simulink model "offline_fuzzypid"  (R2015a)
settings: Solver=ode45  SolverMode=SingleTasking  StartTime=0.0  StopTime=10.0  RelTol=1e-3
libraries: fuzblock x1, simulink x1
settings Model: CovMetricSettings=dwe  CovHtmlReporting=off  covSaveCumulativeToWorkspaceVar=off  CovSaveSingleToWorkspaceVar=off  CovExternalEMLEnable=on  Creator=DwigHT  LastModifiedBy=DwigHT
settings DataIOCC: LimitDataPoints=off  SaveFormat=Dataset  ReturnWorkspaceOutputs=on
settings DebuggingCC: UnconnectedInputMsg=none  UnconnectedOutputMsg=none  UnconnectedLineMsg=none  SFUnexpectedBacktrackingDiag=error  SFNoUnconditionalDefaultTransitionDiag=error
settings HardwareCC: ProdBitPerPointer=64  ProdLargestAtomicFloat=Float  ProdIntDivRoundTo=Zero  ProdEndianess=LittleEndian  ProdHWDeviceType=Specified
settings ModelReferenceCC: PropagateSignalLabelsOutOfModel=on
settings SFSimCC: SimUseLocalCustomCode=on
settings RTWCC: RTWUseLocalCustomCode=on
settings GRTTargetCC: TargetLangStandard=C99 (ISO)

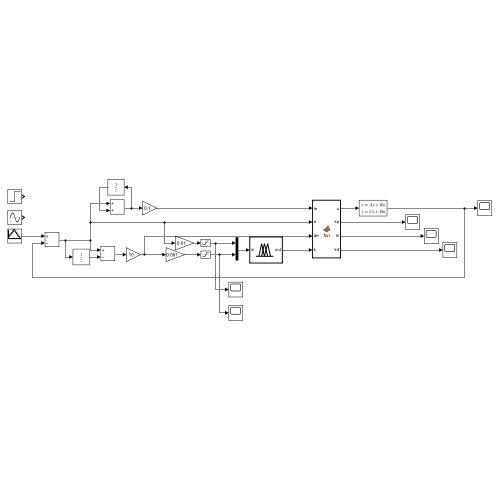
[thumbnail: Simulink's stored preview of the top-level diagram]
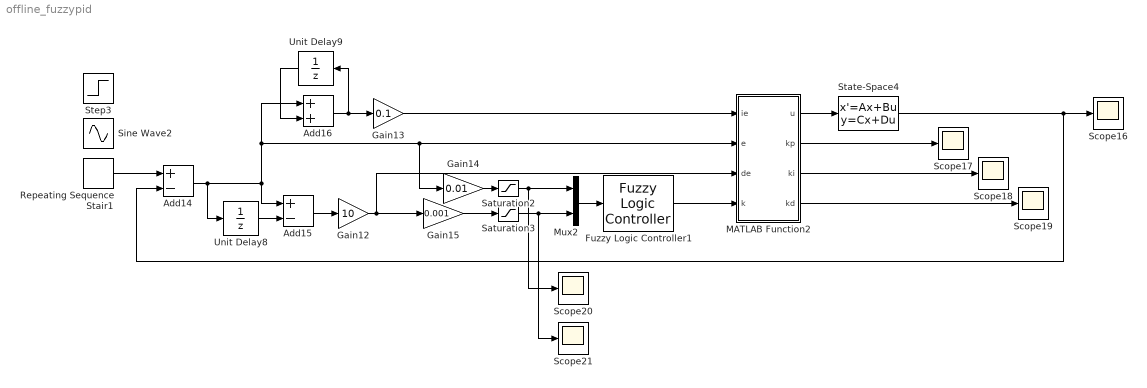
== system offline_fuzzypid ==
  Add14 : Sum  Inputs=+-
  Add15 : Sum  Inputs=+-
  Add16 : Sum
  Fuzzy Logic Controller1 : fuzblock/Fuzzy Logic  Controller  FIS='fuzzpid.fis'
  Gain12 : Gain  Gain=10
  Gain13 : Gain  Gain=0.1
  Gain14 : Gain  Gain=0.01
  Gain15 : Gain  Gain=0.001
  MATLAB Function2 : MATLAB Function  TreatAsAtomicUnit=on
      settings: PermitHierarchicalResolution=ParametersOnly
  Mux2 : Mux  Inputs=2
  Repeating Sequence Stair1 : simulink/Sources/Repeating Sequence Stair  OutValues=[50 100 150 200 150 100 50 0].'  tsamp=5  OutMin=[]  OutMax=[]  OutDataTypeStr=double  OutputDataTypeScalingMode=double  OutDataType=fixdt(0,8)  ConRadixGroup=Best Precision: Vector-wise  OutScaling=2^-12
  Saturation2 : Saturate  UpperLimit=3  LowerLimit=-3
  Saturation3 : Saturate  UpperLimit=3  LowerLimit=-3
  Scope{16..21} (6 alike) : Scope
      Scope16 settings: TimeRange=auto  MaxDataPoints=5000  SaveToWorkspace=off  YMin=-40.57456  YMax=250.19615  SampleTime=-1
      Scope17 settings: TimeRange=auto  MaxDataPoints=5000  SaveToWorkspace=off  SaveName=ScopeData2  YMin=0.21511  YMax=0.30595  SampleTime=-1
      Scope18 settings: TimeRange=auto  MaxDataPoints=5000  SaveToWorkspace=off  SaveName=ScopeData3  YMin=0.63904  YMax=0.80104  SampleTime=-1
      Scope19 settings: TimeRange=auto  MaxDataPoints=5000  SaveToWorkspace=off  SaveName=ScopeData4  YMin=-1.00000  YMax=1.00000  SampleTime=-1
      Scope20 settings: TimeRange=auto  MaxDataPoints=5000  SaveToWorkspace=off  SaveName=ScopeData5  YMin=-10.56926  YMax=2.54153  SampleTime=-1
      Scope21 settings: TimeRange=auto  MaxDataPoints=5000  SaveToWorkspace=off  SaveName=ScopeData6  YMin=-6.54106  YMax=3.28062  SampleTime=-1
  Sine Wave2 : Sin  Amplitude=100  Bias=100  Phase=-pi/2  SampleTime=0
  State-Space4 : StateSpace  A=|  B=|  C="[506.6935  -28.5861   20.0306]"  D=0  X0=0
      A=|
      | [-0.1138    2.9137   -1.5672;
      |    -4.9175   -7.2086    8.0717;
      |     1.4734   -0.1860   -1.7556]
      B=|
      | [   -0.0193;
      |     0.0886;
      |    -0.0121]
  Step3 : Step  After=100  SampleTime=0
  Unit Delay8 : UnitDelay  SampleTime=-1  HasFrameUpgradeWarning=on
  Unit Delay9 : UnitDelay  SampleTime=-1  HasFrameUpgradeWarning=on
  wires:
  Gain12/1 -> MATLAB Function2/3(de), Gain15/1
  Gain15/1 -> Saturation3/1
  Saturation3/1 -> Scope21/1, Mux2/2
  Repeating Sequence Stair1/1 -> Add14/1
  Gain13/1 -> MATLAB Function2/1(ie)
  Add16/1 -> Gain13/1, Unit Delay9/1
  Mux2/1 -> Fuzzy Logic Controller1/1
  MATLAB Function2/3(ki) -> Scope18/1
  Gain14/1 -> Saturation2/1
  MATLAB Function2/4(kd) -> Scope19/1
  Fuzzy Logic Controller1/1 -> MATLAB Function2/4(k)
  Add14/1 -> Add15/1, Add16/1, Gain14/1, MATLAB Function2/2(e), Unit Delay8/1
  Saturation2/1 -> Scope20/1, Mux2/1
  MATLAB Function2/1(u) -> State-Space4/1
  Add15/1 -> Gain12/1
  State-Space4/1 -> Add14/2, Scope16/1
  Unit Delay9/1 -> Add16/2
  MATLAB Function2/2(kp) -> Scope17/1
  Unit Delay8/1 -> Add15/2

== matlab function offline_fuzzypid/MATLAB Function2 ==
  data: ie input; e input; de input; k input; u output; kp output; ki output; kd output
function [u,kp,ki,kd] = fcn(ie,e,de,k)
kp = 0.25+k(1)*1;
ki = 0.72+k(2)*10;
kd = k(3)*0;
u  = kp*e+ki*ie+kd*de;
